simulink model "simulink_ompc"  (R2022b)
settings: Solver=ode5  StartTime=0.0  StopTime=time  FixedStep=Ts  RelTol=1e-3
values from neighbouring files (symbols this model uses):
  A = [A zeros(nA, nAm); zeros(nAm, nA) Am]    [generateBuilding.m]    (also in generateFloor.m; generateRoom.m = [sectionEq;exteriorWallEq;interiorWallEq;roofEq;floorEq]; heatPump.m = -(U*area_buf + m_dot*cw)/C_bufor; mergeFloorModels.m = A0)
  Ao = [Ad Zd; zeros(nz,nx) zeros(nz,nz)]    [plik_generujDane.m]
  B = [B zeros(nA, nBm); zeros(nAm, nB) Bm]    [generateBuilding.m]    (also in generateFloor.m; generateRoom.m = zeros(size(A,1),1); heatPump.m = COP/C_bufor; mergeFloorModels.m = B0)
  Bd = Bd(:, 1:size(B, 2))    [plik_generujDane.m]
  Bo = [Bd; zeros(nz,nu)]    [plik_generujDane.m]
  C = [C zeros(nC, nAm); zeros(nCm, nA) Cm]    [generateBuilding.m]    (also in generateFloor.m; generateRoom.m = [1 0 0 zeros(1,2*n) 0 0 0]; heatPump.m = 1; mergeFloorModels.m = C0)
  Co = [Cd zeros(ny,nz)]    [plik_generujDane.m]
  D = Dm    [generateBuilding.m]    (also in generateFloor.m; generateRoom.m = 0; heatPump.m = 0; mergePumpBuilding.m)
  Go = Go'    [plik_generujDane.m]
  K = P_pred * C' / (C * P_pred * C' + R)    [KalmanFilter.m]
  nc = 20    [plik_generujDane.m]
  npred = 100    [plik_generujDane.m]
  nu = size(B,2)    [ompc_cost.m]    (also in ompc_cost_tracking.m; ompc_law.m; ompc_law_advanced.m; ompc_law_price.m)
  Sc = Spsi(nx+1:end,nx+1:end)    [ompc_cost.m]    (also in ompc_cost_tracking.m = Spsi(nx+1:nx+nuc,nx+1:nx+nuc); ompc_law.m = (Sc+Sc')/2)
  Sx = Spsi(1:nx,1:nx)    [ompc_cost.m]    (also in ompc_cost_tracking.m)
  Sxc = Spsi(1:nx,nx+1:end)    [ompc_cost.m]    (also in ompc_cost_tracking.m = Spsi(1:nx,nx+1:nx+nuc))
  umax = 50*ones(nu,1)    [plik_generujDane.m]
  umin = 0*ones(nu,1)    [plik_generujDane.m]
  x0 = x0'    [initialStates.m]    (also in plik_generujDane.m)
  xmax = [xmax [Ta_max xmax0 Twall_max Twall_max Tp_max T_return_max]]    [initialStates.m]    (also in plik_generujDane.m = xmax')
  xmin = [xmin [Ta_min xmin0 Twall_min Twall_min Tp_min T_return_min]]    [initialStates.m]    (also in plik_generujDane.m = xmin')
  ymax = Ta_max*ones(ny,1)    [plik_generujDane.m]
  ymin = Ta_min*ones(ny,1)    [plik_generujDane.m]
  Z = [Z zeros(nZ, nZmcol-2); Zm(:,1) zeros(nZm, nZcol-2) Zm(:,2:end)]    [generateBuilding.m]    (also in generateFloor.m = [Z zeros(nZ,1); Zm(:,1:2) zeros(nZm,nZcol-2) Zm(:,3)]; generateRoom.m = [0 0 1/Ca; heatPump.m = [U*area_buf m_dot*cw]/C_bufor; mergeFloorModels.m = Z0)
undefined symbols (not defined in the file or in its folder): Ad, Cd
libraries: eeStairGenerator x1, simulink x1
settings Model: Creator=artur  LastModifiedBy=artur

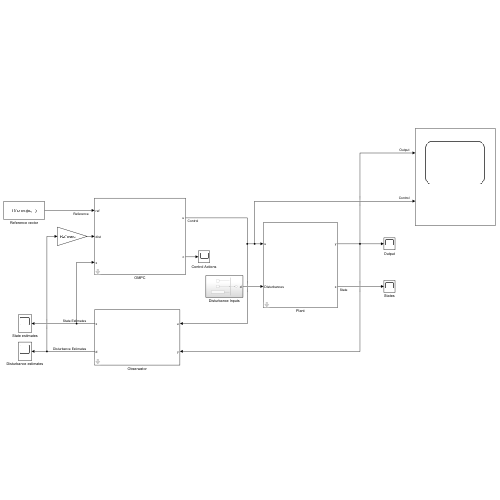
[thumbnail: Simulink's stored preview of the top-level diagram]
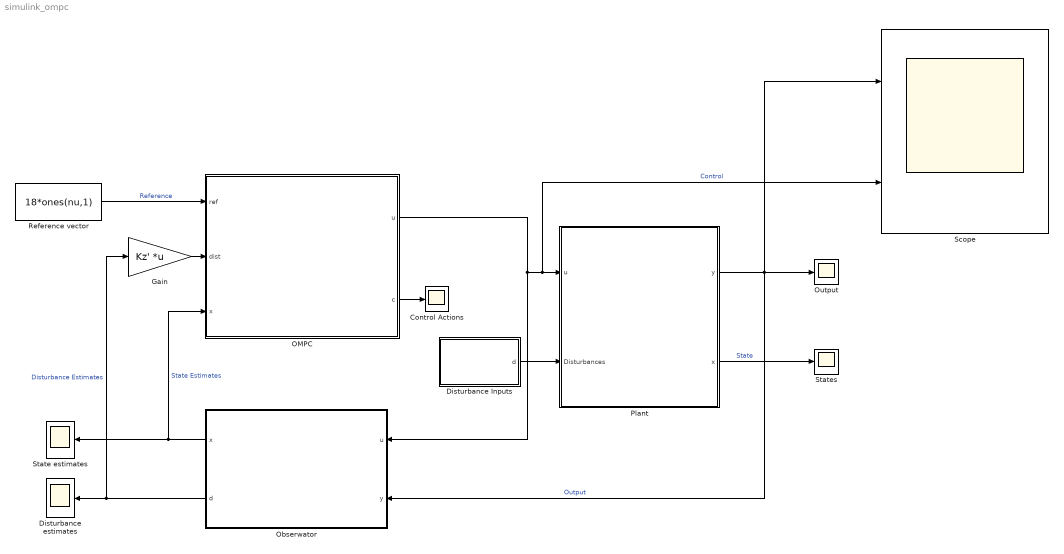
== system simulink_ompc ==
  Control Actions : Scope
  Disturbance Inputs : Subsystem
  Disturbance estimates : Scope
  Gain : Gain  Gain=Kz'  Multiplication=Matrix(K*u) (u vector)
  OMPC : Subsystem  mask{A=Ad, B=Bd, C=Cd, nc=nc, npred=npred, Sx=Sx, Sxc=Sxc, Sc=Sc, K=K, umax=umax, umin=umin, ymax=ymax, ymin=ymin, xmax=xmax, xmin=xmin}
      mask prompts: A "Macierz A"; B "Macierz  B"; C "Macierz C"; nc "Liczba zmiennych decyzyjnych"; npred "Horyzont predykcji"; Sx "Macierz Sx"; Sxc "Macierz Sxc"; Sc "Macierz Sc"; K "Macierz K"
      mask DialogControl ParameterGroupVar Prompt: Parametry modelu
      mask DialogControl Container3 Prompt: Parametry regulatora
      mask DialogControl Container4 Prompt: Ograniczenia
  Obserwator : Subsystem  mask{Ao=Ao, Bo=Bo, Co=Co, Go=Go, A=Ad}
      mask prompts: Ao "Macierz A"; Bo "Macierz B"; Co "Macierz C"; Go "Macierz G"; A "Macierz A modelu"
      mask DialogControl Observer Prompt: Parametry Obserwatora
  Output : Scope
  Plant : Subsystem  mask{A=A, B=B, C=C, D=D, Z=Z, x0=x0}
      mask prompts: A "Macierz A:"; B "Macierz B"; C "Macierz C"; D "Macierz D"; Z "Macierz zakłóceń Z"; x0 "War. początkowe"
      mask DialogControl ParameterGroupVar Prompt: Parametry modelu
  Reference vector : Constant  Value=18*ones(nu,1)
  Scope : Scope  NumInputPorts=2
  State estimates : Scope
  States : Scope
  wires:
  Plant/2(x) -> States/1  "State"
  OMPC/1(u) -> Obserwator/1(u), Plant/1(u), Scope/2  "Control"
  Plant/1(y) -> Obserwator/2(y), Scope/1, Output/1  "Output"
  OMPC/2(c) -> Control Actions/1
  Obserwator/1(x) -> OMPC/3(x), State estimates/1  "State Estimates"
  Obserwator/2(d) -> Gain/1, Disturbance estimates/1  "Disturbance Estimates"
  Reference vector/1 -> OMPC/1(ref)  "Reference"
  Disturbance Inputs/1(d) -> Plant/2(Disturbances)
  Gain/1 -> OMPC/2(dist)

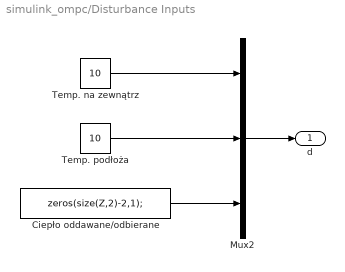
== system simulink_ompc/Disturbance Inputs ==
  Ciepło oddawane/odbierane : Constant  Value=zeros(size(Z,2)-2,1);
  Mux2 : Mux  Inputs=3
  Temp. na zewnątrz : Constant  Value=10
  Temp. podłoża : Constant  Value=10
  d : Outport
  wires:
  Temp. na zewnątrz/1 -> Mux2/1
  Mux2/1 -> d/1
  Ciepło oddawane/odbierane/1 -> Mux2/3
  Temp. podłoża/1 -> Mux2/2

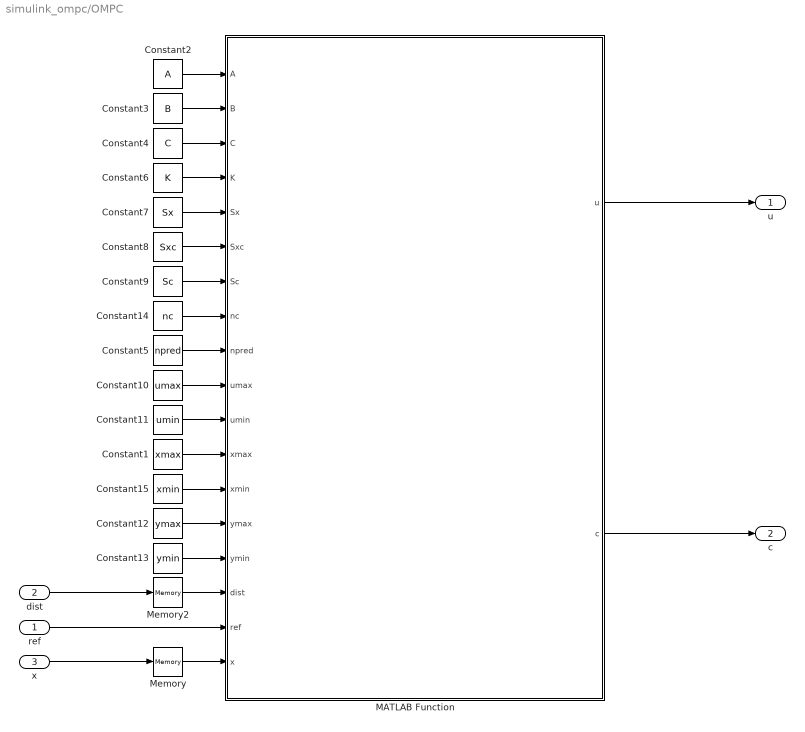
== system simulink_ompc/OMPC ==
  ref : Inport
  dist : Inport  Port=2
  x : Inport  Port=3
  Constant1 : Constant  Value=xmax  VectorParams1D=off
  Constant10 : Constant  Value=umax  VectorParams1D=off
  Constant11 : Constant  Value=umin  VectorParams1D=off
  Constant12 : Constant  Value=ymax
  Constant13 : Constant  Value=ymin
  Constant14 : Constant  Value=nc
  Constant15 : Constant  Value=xmin
  Constant2 : Constant  Value=A
  Constant3 : Constant  Value=B  VectorParams1D=off
  Constant4 : Constant  Value=C  VectorParams1D=off
  Constant5 : Constant  Value=npred
  Constant6 : Constant  Value=K  VectorParams1D=off
  Constant7 : Constant  Value=Sx  VectorParams1D=off
  Constant8 : Constant  Value=Sxc  VectorParams1D=off
  Constant9 : Constant  Value=Sc  VectorParams1D=off
  MATLAB Function : MATLAB Function  TreatAsAtomicUnit=on
  Memory : Memory  InitialCondition=x0
  Memory2 : Memory  InitialCondition=zeros(size(C,1),1)
  u : Outport
  c : Outport  Port=2
  wires:
  Constant6/1 -> MATLAB Function/4(K)
  Constant9/1 -> MATLAB Function/7(Sc)
  Constant8/1 -> MATLAB Function/6(Sxc)
  Constant2/1 -> MATLAB Function/1(A)
  Constant7/1 -> MATLAB Function/5(Sx)
  Constant4/1 -> MATLAB Function/3(C)
  x/1 -> Memory/1
  Constant3/1 -> MATLAB Function/2(B)
  ref/1 -> MATLAB Function/17(ref)
  Constant10/1 -> MATLAB Function/10(umax)
  Constant11/1 -> MATLAB Function/11(umin)
  Constant12/1 -> MATLAB Function/14(ymax)
  Constant13/1 -> MATLAB Function/15(ymin)
  Memory/1 -> MATLAB Function/18(x)
  dist/1 -> Memory2/1
  MATLAB Function/2(c) -> c/1
  Constant5/1 -> MATLAB Function/9(npred)
  Constant14/1 -> MATLAB Function/8(nc)
  Memory2/1 -> MATLAB Function/16(dist)
  Constant15/1 -> MATLAB Function/13(xmin)
  Constant1/1 -> MATLAB Function/12(xmax)
  MATLAB Function/1(u) -> u/1

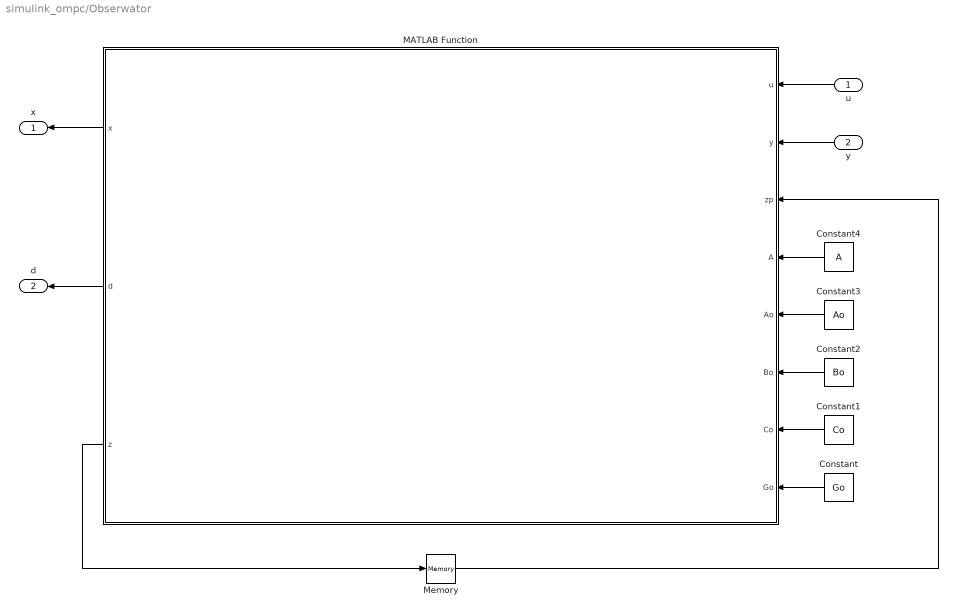
== system simulink_ompc/Obserwator ==
  u : Inport
  y : Inport  Port=2
  Constant : Constant  Value=Go  VectorParams1D=off
  Constant1 : Constant  Value=Co  VectorParams1D=off
  Constant2 : Constant  Value=Bo  VectorParams1D=off
  Constant3 : Constant  Value=Ao  VectorParams1D=off
  Constant4 : Constant  Value=A
  MATLAB Function : MATLAB Function  TreatAsAtomicUnit=on
  Memory : Memory  InitialCondition=[x0;zeros(size(Z,2),1)]
  x : Outport
  d : Outport  Port=2
  wires:
  Constant3/1 -> MATLAB Function/5(Ao)
  Constant1/1 -> MATLAB Function/7(Co)
  Constant2/1 -> MATLAB Function/6(Bo)
  Constant/1 -> MATLAB Function/8(Go)
  Memory/1 -> MATLAB Function/3(zp)
  y/1 -> MATLAB Function/2(y)
  u/1 -> MATLAB Function/1(u)
  MATLAB Function/3(z) -> Memory/1
  MATLAB Function/1(x) -> x/1
  MATLAB Function/2(d) -> d/1
  Constant4/1 -> MATLAB Function/4(A)

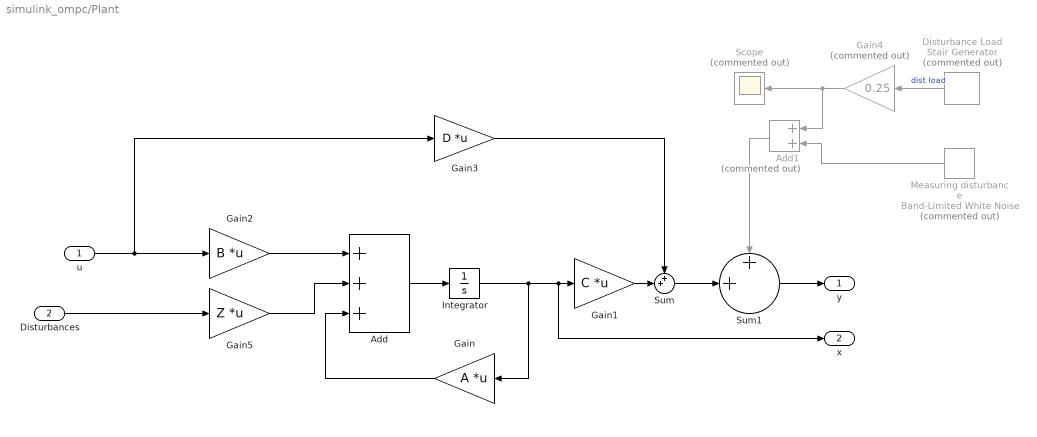
== system simulink_ompc/Plant ==
  u : Inport
  Disturbances : Inport  Port=2
  Add : Sum  Inputs=+++
  Add1 : Sum  Commented=on
  Disturbance Load : eeStairGenerator/Stair Generator  Commented=on  LabelModeActiveChoice=Discrete  TimeInput=[0 5 10 15 20 25 30 35 40 45 50]  AmplitudeInput=[1 1 1 -1 -1 -1 1 1 -1 -1 1]  SampleTime=0.1  RepeatPattern=on  OutDataTypeStr=double
      settings: LibrarySourceBlock=ee_sl_lib/General Control/Stair Generator
  Gain : Gain  Gain=A  Multiplication=Matrix(K*u) (u vector)
  Gain1 : Gain  Gain=C  Multiplication=Matrix(K*u) (u vector)
  Gain2 : Gain  Gain=B  Multiplication=Matrix(K*u) (u vector)
  Gain3 : Gain  Gain=D  Multiplication=Matrix(K*u)
  Gain4 : Gain  Commented=on  Gain=0.25
  Gain5 : Gain  Gain=Z  Multiplication=Matrix(K*u) (u vector)
  Integrator : Integrator  InitialCondition=x0
  Measuring disturbance : simulink/Sources/Band-Limited White Noise  Commented=on  Cov=[0.002]  Ts=0.1  seed=[23341]
  Scope : Scope  Commented=on
  Sum : Sum  Inputs=++|
  Sum1 : Sum  Inputs=++|
  y : Outport
  x : Outport  Port=2
  wires:
  u/1 -> Gain3/1, Gain2/1
  Integrator/1 -> x/1, Gain1/1, Gain/1
  Add/1 -> Integrator/1
  Gain2/1 -> Add/1
  Gain1/1 -> Sum/2
  Gain3/1 -> Sum/1
  Sum1/1 -> y/1
  Sum/1 -> Sum1/2
  Disturbance Load/1 -> Gain4/1  "dist load"
  Add1/1 -> Sum1/1
  Measuring disturbance/1 -> Add1/2
  Gain4/1 -> Add1/1, Scope/1
  Gain/1 -> Add/3
  Disturbances/1 -> Gain5/1
  Gain5/1 -> Add/2

== matlab function simulink_ompc/Obserwator/MATLAB Function ==
  data: u input; x output; y input; zp input; A input; Ao input; Bo input; Co input; Go input; d output; z output
function [x,d,z] = fcn(u,y,zp,A,Ao,Bo,Co,Go)

nx = size(A,1);
z = Ao*zp + Bo*u + Go*(y - Co*zp);
x = z(1:nx,:);
d = z(nx+1:end,:);

== matlab function simulink_ompc/OMPC/MATLAB Function ==
  data: A input; B input; C input; K input; Sx input; Sxc input; Sc input; nc input; npred input; umax input; umin input; xmax input; xmin input; ymax input; ymin input; dist input; ref input; x input; u output; c output
function [u,c] = fcn(A,B,C,K,Sx,Sxc,Sc,nc,npred,umax,umin,xmax,xmin,ymax,ymin,dist,ref,x)

% [u,c] = ompc_law_unconstrained(A,B,C,K,Sx,Sxc,Sc,ref,dist,x);
[u,ctrl] = ompc_law(A,B,C,K,Sx,Sxc,Sc,umax,umin,xmax,xmin,ymax,ymin,nc,npred,ref,dist,x);
c = ctrl(1:size(B,2),:);
